simulink model "joint_space_inv_dyn"  (R2020b)
settings: Solver=FixedStepAuto  StartTime=0.0  StopTime=10  FixedStep=Ts  RelTol=1e-3
values from neighbouring files (symbols this model uses):
  dqi = [0 0 0]'    [main_3DoF_robots.m]
  he = [fex fey fez uex uey uez]'    [MyRobot.m]    (also in getBHat.m = zeros(6,1); main_3DoF_robots.m = [0 0 0 0 0 0]')
  Kd_inv = [10;5;10]    [main_3DoF_robots.m]
  Kp_inv = [50;100;50]    [main_3DoF_robots.m]
  myRobot = MyRobot('PRP.urdf', DH, links)    [main_3DoF_robots.m]
  qi = [0 0 0]'    [main_3DoF_robots.m]
settings Model: Creator=simon  LastModifiedBy=SimoneCremasco
settings SolverCC: ZeroCrossControl=DisableAll

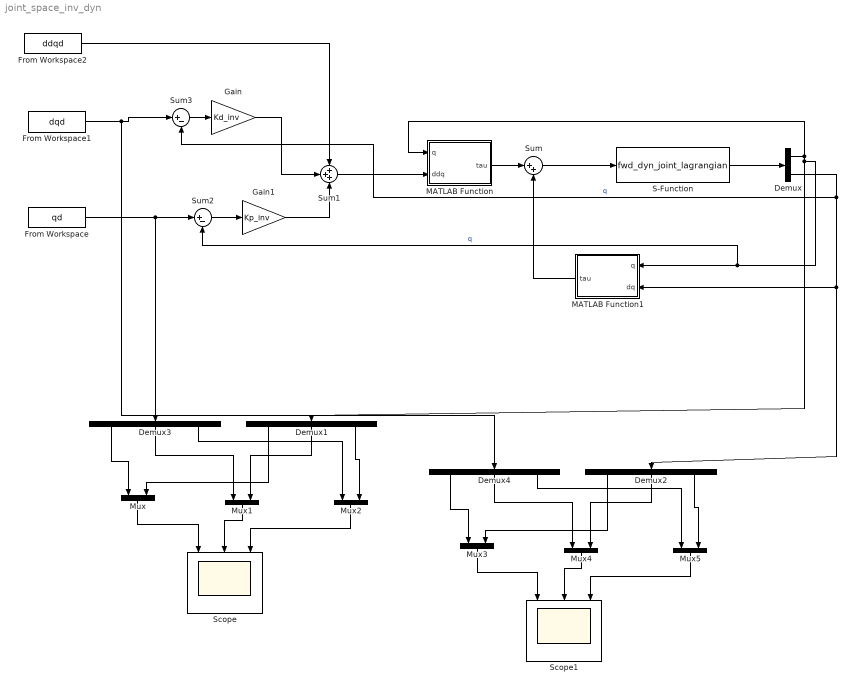
== system joint_space_inv_dyn ==
  Demux : Demux  Outputs=2
  Demux{1..4} (4 alike) : Demux  Outputs=myRobot.N
  From Workspace : FromWorkspace  VariableName=qd
  From Workspace1 : FromWorkspace  VariableName=dqd
  From Workspace2 : FromWorkspace  VariableName=ddqd
  Gain : Gain  Gain=Kd_inv
  Gain1 : Gain  Gain=Kp_inv
  MATLAB Function : MATLAB Function  TreatAsAtomicUnit=on
  MATLAB Function1 : MATLAB Function  TreatAsAtomicUnit=on
  Mux{,1..5} (6 alike) : Mux  Inputs=2
  S-Function : S-Function  FunctionName=fwd_dyn_joint_lagrangian  Parameters=myRobot,he,qi,dqi  SFunctionDeploymentMode=off  EnableBusSupport=off
  Scope : Scope  NumInputPorts=3
  Scope1 : Scope  NumInputPorts=3
  Sum : Sum  Inputs=|++
  Sum1 : Sum  Inputs=+++
  Sum2 : Sum  Inputs=|+-
  Sum3 : Sum  Inputs=|+-
  wires:
  S-Function/1 -> Demux/1
  MATLAB Function/1(tau) -> Sum/1
  MATLAB Function1/1(tau) -> Sum/2
  Sum/1 -> S-Function/1
  Sum1/1 -> MATLAB Function/2(ddq)
  Gain1/1 -> Sum1/3
  Gain/1 -> Sum1/2
  Sum3/1 -> Gain/1
  Sum2/1 -> Gain1/1
  From Workspace2/1 -> Sum1/1
  Mux1/1 -> Scope/2
  From Workspace/1 -> Sum2/1, Demux3/1
  Mux2/1 -> Scope/3
  Demux1/3 -> Mux2/2
  Mux/1 -> Scope/1
  Demux1/2 -> Mux1/2
  Demux1/1 -> Mux/2
  Demux3/1 -> Mux/1
  Demux/1 -> Demux1/1, Sum2/2, MATLAB Function1/1(q), MATLAB Function/1(q)  "q"
  Demux3/2 -> Mux1/1
  Demux3/3 -> Mux2/1
  Demux/2 -> Sum3/2, Demux2/1, MATLAB Function1/2(dq)  "q"
  Demux4/2 -> Mux4/1
  Demux4/3 -> Mux5/1
  Demux4/1 -> Mux3/1
  Mux5/1 -> Scope1/3
  Mux3/1 -> Scope1/1
  Demux2/3 -> Mux5/2
  Mux4/1 -> Scope1/2
  Demux2/1 -> Mux3/2
  From Workspace1/1 -> Demux4/1, Sum3/1
  Demux2/2 -> Mux4/2

== matlab function joint_space_inv_dyn/MATLAB Function ==
  data: q input size=3; tau output; ddq input size=3
function tau = B(q, ddq)

tau = getB(q)*ddq;

== matlab function joint_space_inv_dyn/MATLAB Function1 ==
  data: q input size=3; tau output; dq input size=3
function tau = fcn(q, dq)

tau = getN(q, dq);
